simulink subsystem "IFCamera"  (R2025a)
settings: Solver=VariableStepAuto  StartTime=0.0  StopTime=10.0  RelTol=1e-3
settings Model: Creator=yvijay  LastModifiedBy=atcushen

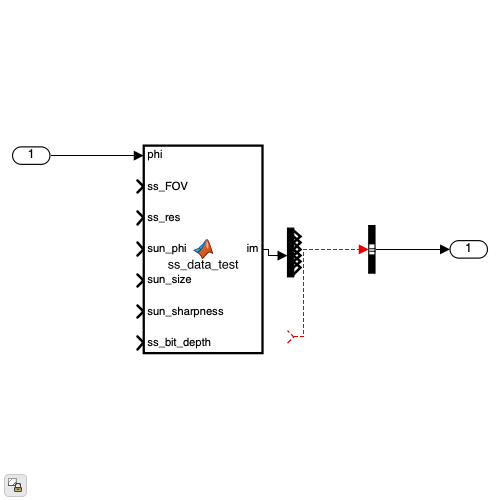
[thumbnail: Simulink's stored preview of the top-level diagram]
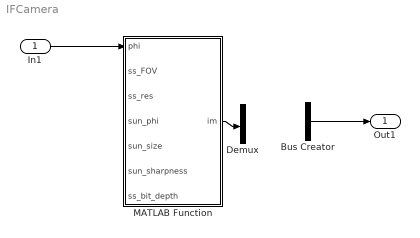
== system IFCamera ==
  In1 : Inport
  Bus Creator : BusCreator  Inputs=1
  Demux : Demux  Outputs=6
  MATLAB Function : MATLAB Function  TreatAsAtomicUnit=on
  Out1 : Outport
  wires:
  In1/1 -> MATLAB Function/1(phi)
  MATLAB Function/1(im) -> Demux/1
  Bus Creator/1 -> Out1/1
  ? -> Bus Creator/1

== matlab function IFCamera/MATLAB Function ==
  data: phi input; im output; ss_FOV input; ss_res input; sun_phi input; sun_size input; sun_sharpness input; ss_bit_depth input
function im = ss_data_test(phi,ss_FOV,ss_res,sun_phi,sun_size,sun_sharpness,ss_bit_depth)
    %im = zeros(ss_res, ss_res); % Initialize image array as zeros

    phi_ax = linspace(phi-ss_FOV,phi+ss_FOV,ss_res); % Determine phi axis of image
    theta_ax = linspace(-ss_FOV,ss_FOV,ss_res); % Determine theta axis of image

    [phi_im, theta_im] = meshgrid(phi_ax, theta_ax); % Create 2D array of angle coordinates
    im = ss_bit_depth * exp(-((((phi_im-sun_phi).^2+theta_im.^2)/sun_size^2).^sun_sharpness));
end
